simulink model "IEEE9Buses"  (R2024b)
settings: Solver=FixedStepAuto  StartTime=0  StopTime=5  FixedStep=1e-6  RelTol=1e-3
values from neighbouring files (symbols this model uses):
  SG_D_1_D = 0.01056    [SG9_parameters.m]
  SG_D_1_EnableSaturation = 0    [SG9_parameters.m]
  SG_D_1_f0 = 60    [SG9_parameters.m]
  SG_D_1_H = 7.5    [SG9_parameters.m]
  SG_D_1_K_A = 20    [SG9_parameters.m]
  SG_D_1_K_E = 1.000000e+1    (= 10)    [SG9_parameters.m]
  SG_D_1_K_F = 2.363    [SG9_parameters.m]
  SG_D_1_K_s = 5    [SG9_parameters.m]
  SG_D_1_R_a = 0.001088    [SG9_parameters.m]
  SG_D_1_S_A = 1    [SG9_parameters.m]
  SG_D_1_S_B = 0.103    [SG9_parameters.m]
  SG_D_1_S_N = 10.659857    [SG9_parameters.m]
  SG_D_1_SpeedPara = 200    [SG9_parameters.m]
  SG_D_1_T_0 = 0.720173    [SG9_parameters.m]
  SG_D_1_T_1 = 0.3    [SG9_parameters.m]
  SG_D_1_T_2 = 0.05    [SG9_parameters.m]
  SG_D_1_T_3 = 0.02    [SG9_parameters.m]
  SG_D_1_T_4 = 0.005    [SG9_parameters.m]
  SG_D_1_T_A = 0.02    [SG9_parameters.m]
  SG_D_1_T_dd = 8.000000e+0    (= 8)    [SG9_parameters.m]
  SG_D_1_T_ddd = 0.04    [SG9_parameters.m]
  SG_D_1_T_E = 0.314    [SG9_parameters.m]
  SG_D_1_T_F = 0.35    [SG9_parameters.m]
  SG_D_1_T_qd = 0.8    [SG9_parameters.m]
  SG_D_1_T_qdd = 0.02    [SG9_parameters.m]
  SG_D_1_T_speed = 0.1    [SG9_parameters.m]
  SG_D_1_T_w = 0.5    [SG9_parameters.m]
  SG_D_1_V_ref = 1.990276    [SG9_parameters.m]
  SG_D_1_w_ref = 376.991118    [SG9_parameters.m]
  SG_D_1_x_d = 1.9    [SG9_parameters.m]
  SG_D_1_x_dd = 0.302    [SG9_parameters.m]
  SG_D_1_x_ddd = 0.204    [SG9_parameters.m]
  SG_D_1_x_l = 0.05    [SG9_parameters.m]
  SG_D_1_x_q = 1.3    [SG9_parameters.m]
  SG_D_1_x_qd = 0.5    [SG9_parameters.m]
  SG_D_1_x_qdd = 0.3    [SG9_parameters.m]
  SG_D_2_D = 0.01056    [SG9_parameters.m]
  SG_D_2_EnableSaturation = 0    [SG9_parameters.m]
  SG_D_2_f0 = 60    [SG9_parameters.m]
  SG_D_2_H = 7.5    [SG9_parameters.m]
  SG_D_2_K_A = 20    [SG9_parameters.m]
  SG_D_2_K_E = 1.000000e+1    (= 10)    [SG9_parameters.m]
  SG_D_2_K_F = 2.363    [SG9_parameters.m]
  SG_D_2_K_s = 0.5    [SG9_parameters.m]
  SG_D_2_R_a = 0.001088    [SG9_parameters.m]
  SG_D_2_S_A = 1    [SG9_parameters.m]
  SG_D_2_S_B = 0.103    [SG9_parameters.m]
  SG_D_2_S_N = 10.659857    [SG9_parameters.m]
  SG_D_2_SpeedPara = 200    [SG9_parameters.m]
  SG_D_2_T_0 = 1.632913    [SG9_parameters.m]
  SG_D_2_T_1 = 0.2    [SG9_parameters.m]
  SG_D_2_T_2 = 0.05    [SG9_parameters.m]
  SG_D_2_T_3 = 0.02    [SG9_parameters.m]
  SG_D_2_T_4 = 0.005    [SG9_parameters.m]
  SG_D_2_T_A = 0.02    [SG9_parameters.m]
  SG_D_2_T_dd = 8.000000e+0    (= 8)    [SG9_parameters.m]
  SG_D_2_T_ddd = 0.04    [SG9_parameters.m]
  SG_D_2_T_E = 0.314    [SG9_parameters.m]
  SG_D_2_T_F = 0.35    [SG9_parameters.m]
  SG_D_2_T_qd = 0.8    [SG9_parameters.m]
  SG_D_2_T_qdd = 0.02    [SG9_parameters.m]
  SG_D_2_T_speed = 0.1    [SG9_parameters.m]
  SG_D_2_T_w = 0.5    [SG9_parameters.m]
  SG_D_2_V_ref = 2.662631    [SG9_parameters.m]
  SG_D_2_w_ref = 376.991118    [SG9_parameters.m]
  SG_D_2_x_d = 1.9    [SG9_parameters.m]
  SG_D_2_x_dd = 0.302    [SG9_parameters.m]
  SG_D_2_x_ddd = 0.204    [SG9_parameters.m]
  SG_D_2_x_l = 0.05    [SG9_parameters.m]
  SG_D_2_x_q = 1.3    [SG9_parameters.m]
  SG_D_2_x_qd = 0.5    [SG9_parameters.m]
  SG_D_2_x_qdd = 0.3    [SG9_parameters.m]
  SG_D_3_D = 0.01056    [SG9_parameters.m]
  SG_D_3_EnableSaturation = 0    [SG9_parameters.m]
  SG_D_3_f0 = 60    [SG9_parameters.m]
  SG_D_3_H = 7.5    [SG9_parameters.m]
  SG_D_3_K_A = 20    [SG9_parameters.m]
  SG_D_3_K_E = 1.000000e+1    (= 10)    [SG9_parameters.m]
  SG_D_3_K_F = 2.363    [SG9_parameters.m]
  SG_D_3_K_s = 0.5    [SG9_parameters.m]
  SG_D_3_R_a = 0.001088    [SG9_parameters.m]
  SG_D_3_S_A = 1    [SG9_parameters.m]
  SG_D_3_S_B = 0.103    [SG9_parameters.m]
  SG_D_3_S_N = 10.659857    [SG9_parameters.m]
  SG_D_3_SpeedPara = 200    [SG9_parameters.m]
  SG_D_3_T_0 = 0.850788    [SG9_parameters.m]
  SG_D_3_T_1 = 0.2    [SG9_parameters.m]
  SG_D_3_T_2 = 0.05    [SG9_parameters.m]
  SG_D_3_T_3 = 0.02    [SG9_parameters.m]
  SG_D_3_T_4 = 0.005    [SG9_parameters.m]
  SG_D_3_T_A = 0.02    [SG9_parameters.m]
  SG_D_3_T_dd = 8.000000e+0    (= 8)    [SG9_parameters.m]
  SG_D_3_T_ddd = 0.04    [SG9_parameters.m]
  SG_D_3_T_E = 0.314    [SG9_parameters.m]
  SG_D_3_T_F = 0.35    [SG9_parameters.m]
  SG_D_3_T_qd = 0.8    [SG9_parameters.m]
  SG_D_3_T_qdd = 0.02    [SG9_parameters.m]
  SG_D_3_T_speed = 0.1    [SG9_parameters.m]
  SG_D_3_T_w = 0.5    [SG9_parameters.m]
  SG_D_3_V_ref = 1.915682    [SG9_parameters.m]
  SG_D_3_w_ref = 376.991118    [SG9_parameters.m]
  SG_D_3_x_d = 1.9    [SG9_parameters.m]
  SG_D_3_x_dd = 0.302    [SG9_parameters.m]
  SG_D_3_x_ddd = 0.204    [SG9_parameters.m]
  SG_D_3_x_l = 0.05    [SG9_parameters.m]
  SG_D_3_x_q = 1.3    [SG9_parameters.m]
  SG_D_3_x_qd = 0.5    [SG9_parameters.m]
  SG_D_3_x_qdd = 0.3    [SG9_parameters.m]
(part 5 of 9)

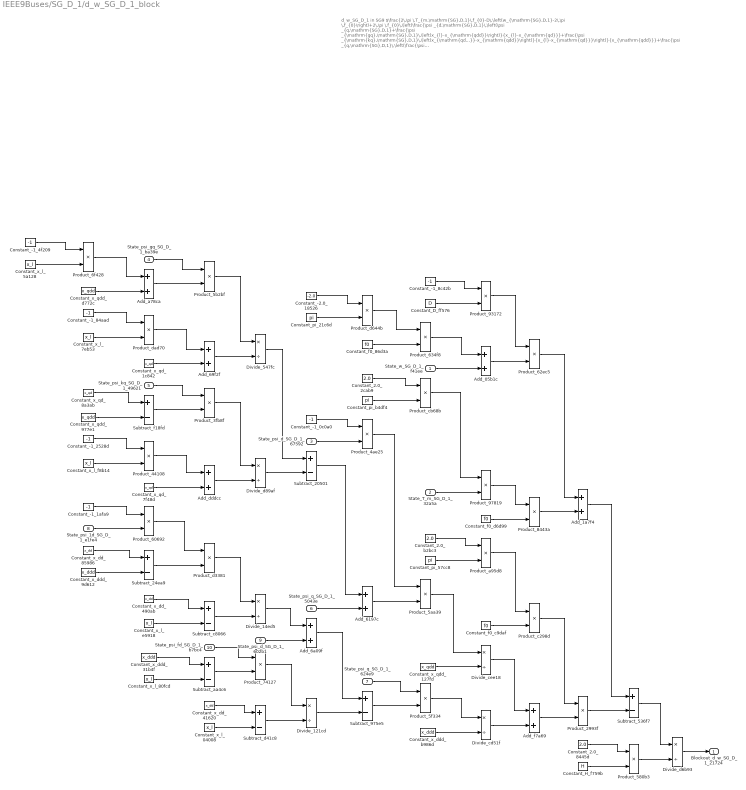
== system IEEE9Buses/SG_D_1/d_w_SG_D_1_block ==
  note: d_w_SG_D_1 in SG9
      | $\frac{2\,\pi \,T_{m,\mathrm{SG},D,1}\,f_{0}-D\,\left(w_{\mathrm{SG},D,1}-2\,\pi \,f_{0}\right)+2\,\pi \,f_{0}\,\left(\frac{\psi _{d,\mathrm{SG},D,1}\,\left(\psi _{q,\mathrm{SG},D,1}+\frac{\psi _{\mathrm{gq},\mathrm{SG},D,1}\,\left(x_{l}-x_{\mathrm{qdd}}\right)}{x_{l}-x_{\mathrm{qd}}}+\frac{\psi _{\mathrm{kq},\mathrm{SG},D,1}\,\left(x_{\mathrm{qd}}-x_{\mathrm{qdd}}\right)}{x_{l}-x_{\mathrm{qd}}}\right)}{x_{\mathrm{qdd}}}+\frac{\psi _{q,\mathrm{SG},D,1}\,\left(\frac{\psi _{\mathrm{1d},\mathrm{SG},D,1}\,\left(x_{\mathrm{dd}}-x_{\mathrm{ddd}}\right)}{x_{\mathrm{dd}}-x_{l}}-\psi _{d,\mathrm{SG},D,1}+\frac{\psi _{\mathrm{fd},\mathrm{SG},D,1}\,\left(x_{\mathrm{ddd}}-x_{l}\right)}{x_{\mathrm{dd}}-x_{l}}\right)}{x_{\mathrm{ddd}}}\right)}{2\,H}$
      | Automatically generated on 2025-09-12 21:31:18 .
  State_w_SG_D_1_f41ee : Inport
  State_T_m_SG_D_1_32a5a : Inport  Port=2
  State_psi_d_SG_D_1_67592 : Inport  Port=3
  State_psi_gq_SG_D_1_ba39e : Inport  Port=4
  State_psi_kq_SG_D_1_49621 : Inport  Port=5
  State_psi_q_SG_D_1_5043e : Inport  Port=6
  State_psi_q_SG_D_1_624e9 : Inport  Port=7
  State_psi_1d_SG_D_1_e1fe4 : Inport  Port=8
  State_psi_d_SG_D_1_602b1 : Inport  Port=9
  State_psi_fd_SG_D_1_b7bc4 : Inport  Port=10
  Add_05b1c : Sum
  Add_1a7f4 : Sum
  Add_6197c : Sum
  Add_69f2f : Sum
  Add_6a09f : Sum
  Add_a78ca : Sum
  Add_dddcc : Sum
  Add_f7a69 : Sum
  Constant_-1_0c0a0 : Constant  Value=-1
  Constant_-1_1afa9 : Constant  Value=-1
  Constant_-1_2528d : Constant  Value=-1
  Constant_-1_4f209 : Constant  Value=-1
  Constant_-1_84aad : Constant  Value=-1
  Constant_-1_8c42b : Constant  Value=-1
  Constant_-2.0_18526 : Constant  Value=-2.0
  Constant_2.0_2cab9 : Constant  Value=2.0
  Constant_2.0_8445d : Constant  Value=2.0
  Constant_2.0_b2bc3 : Constant  Value=2.0
  Constant_D_ff576 : Constant  Value=D
  Constant_H_f759b : Constant  Value=H
  Constant_f0_86d3a : Constant  Value=f0
  Constant_f0_c9daf : Constant  Value=f0
  Constant_f0_d6d99 : Constant  Value=f0
  Constant_pi_21c6d : Constant  Value=pi
  Constant_pi_57cc8 : Constant  Value=pi
  Constant_pi_b4df4 : Constant  Value=pi
  Constant_x_dd_41620 : Constant  Value=x_dd
  Constant_x_dd_490ab : Constant  Value=x_dd
  Constant_x_dd_85986 : Constant  Value=x_dd
  Constant_x_ddd_31b4f : Constant  Value=x_ddd
  Constant_x_ddd_9d612 : Constant  Value=x_ddd
  Constant_x_ddd_b986d : Constant  Value=x_ddd
  Constant_x_l_04008 : Constant  Value=x_l
  Constant_x_l_5a128 : Constant  Value=x_l
  Constant_x_l_7eb53 : Constant  Value=x_l
  Constant_x_l_80fcd : Constant  Value=x_l
  Constant_x_l_e5918 : Constant  Value=x_l
  Constant_x_l_f8b14 : Constant  Value=x_l
  Constant_x_qd_1c842 : Constant  Value=x_qd
  Constant_x_qd_7f48d : Constant  Value=x_qd
  Constant_x_qd_8a3ab : Constant  Value=x_qd
  Constant_x_qdd_127fd : Constant  Value=x_qdd
  Constant_x_qdd_977e1 : Constant  Value=x_qdd
  Constant_x_qdd_d772c : Constant  Value=x_qdd
  Divide_121cd : Product  Inputs=*/
  Divide_14ed5 : Product  Inputs=*/
  Divide_547fc : Product  Inputs=*/
  Divide_cd51f : Product  Inputs=*/
  Divide_cee18 : Product  Inputs=*/
  Divide_d6b93 : Product  Inputs=*/
  Divide_d89af : Product  Inputs=*/
  Product_2993f : Product
  Product_3fb8f : Product
  Product_{44108,60692,74127,93172,97819} (5 alike) : Product
  Product_4ae25 : Product
  Product_580b3 : Product
  Product_5aa39 : Product
  Product_5b2bf : Product
  Product_5f334 : Product
  Product_62ec5 : Product
  Product_634f8 : Product
  Product_6f428 : Product
  Product_8443a : Product
  Product_a95d8 : Product
  Product_c298d : Product
  Product_cb68b : Product
  Product_d3381 : Product
  Product_d644b : Product
  Product_dad70 : Product
  Subtract_20501 : Sum  Inputs=+-
  Subtract_24ea9 : Sum  Inputs=+-
  Subtract_536f7 : Sum  Inputs=+-
  Subtract_975e5 : Sum  Inputs=+-
  Subtract_aa4c6 : Sum  Inputs=+-
  Subtract_c8066 : Sum  Inputs=+-
  Subtract_d41c8 : Sum  Inputs=+-
  Subtract_f18fd : Sum  Inputs=+-
  Blockout_d_w_SG_D_1_21724 : Outport
  wires:
  Product_634f8/1 -> Add_05b1c/1
  Constant_-1_4f209/1 -> Product_6f428/1
  Constant_pi_b4df4/1 -> Product_cb68b/2
  Constant_x_qdd_d772c/1 -> Add_a78ca/2
  Constant_x_l_5a128/1 -> Product_6f428/2
  Product_6f428/1 -> Add_a78ca/1
  Constant_x_qd_8a3ab/1 -> Subtract_f18fd/1
  Constant_-1_84aad/1 -> Product_dad70/1
  Product_d644b/1 -> Product_634f8/1
  Constant_x_qdd_977e1/1 -> Subtract_f18fd/2
  State_psi_q_SG_D_1_624e9/1 -> Product_5f334/1
  Constant_x_l_7eb53/1 -> Product_dad70/2
  Constant_-1_2528d/1 -> Product_44108/1
  Constant_x_l_f8b14/1 -> Product_44108/2
  Constant_-1_1afa9/1 -> Product_60692/1
  Product_dad70/1 -> Add_69f2f/1
  State_psi_1d_SG_D_1_e1fe4/1 -> Product_60692/2
  Constant_x_dd_85986/1 -> Subtract_24ea9/1
  Subtract_f18fd/1 -> Product_3fb8f/2
  Constant_x_ddd_9d612/1 -> Subtract_24ea9/2
  State_psi_gq_SG_D_1_ba39e/1 -> Product_5b2bf/1
  Product_4ae25/1 -> Product_5aa39/1
  Add_a78ca/1 -> Product_5b2bf/2
  Constant_x_qd_1c842/1 -> Add_69f2f/2
  State_psi_kq_SG_D_1_49621/1 -> Product_3fb8f/1
  Constant_f0_86d3a/1 -> Product_634f8/2
  Product_44108/1 -> Add_dddcc/1
  Constant_x_dd_490ab/1 -> Subtract_c8066/1
  Constant_x_qd_7f48d/1 -> Add_dddcc/2
  Product_60692/1 -> Product_d3381/1
  Subtract_24ea9/1 -> Product_d3381/2
  Constant_x_l_e5918/1 -> Subtract_c8066/2
  Constant_x_ddd_31b4f/1 -> Subtract_aa4c6/1
  Constant_x_l_80fcd/1 -> Subtract_aa4c6/2
  State_w_SG_D_1_f41ee/1 -> Add_05b1c/2
  Divide_cee18/1 -> Add_f7a69/1
  Constant_-1_8c42b/1 -> Product_93172/1
  Product_5b2bf/1 -> Divide_547fc/1
  Add_05b1c/1 -> Product_62ec5/2
  Divide_547fc/1 -> Subtract_20501/1
  Add_69f2f/1 -> Divide_547fc/2
  Constant_pi_21c6d/1 -> Product_d644b/2
  Product_3fb8f/1 -> Divide_d89af/1
  Add_dddcc/1 -> Divide_d89af/2
  Product_d3381/1 -> Divide_14ed5/1
  Divide_14ed5/1 -> Add_6a09f/1
  Subtract_c8066/1 -> Divide_14ed5/2
  State_psi_fd_SG_D_1_b7bc4/1 -> Product_74127/1
  Subtract_aa4c6/1 -> Product_74127/2
  Constant_x_dd_41620/1 -> Subtract_d41c8/1
  Constant_x_l_04008/1 -> Subtract_d41c8/2
  Divide_d89af/1 -> Subtract_20501/2
  Constant_2.0_2cab9/1 -> Product_cb68b/1
  State_psi_d_SG_D_1_602b1/1 -> Add_6a09f/2
  Product_74127/1 -> Divide_121cd/1
  Subtract_d41c8/1 -> Divide_121cd/2
  Constant_-2.0_18526/1 -> Product_d644b/1
  Constant_-1_0c0a0/1 -> Product_4ae25/1
  State_psi_d_SG_D_1_67592/1 -> Product_4ae25/2
  Subtract_20501/1 -> Add_6197c/1
  Subtract_975e5/1 -> Product_5f334/2
  State_psi_q_SG_D_1_5043e/1 -> Add_6197c/2
  Add_6a09f/1 -> Subtract_975e5/1
  Divide_121cd/1 -> Subtract_975e5/2
  Add_6197c/1 -> Product_5aa39/2
  Constant_D_ff576/1 -> Product_93172/2
  Product_cb68b/1 -> Product_97819/1
  State_T_m_SG_D_1_32a5a/1 -> Product_97819/2
  Constant_2.0_b2bc3/1 -> Product_a95d8/1
  Constant_pi_57cc8/1 -> Product_a95d8/2
  Product_5aa39/1 -> Divide_cee18/1
  Constant_x_qdd_127fd/1 -> Divide_cee18/2
  Product_5f334/1 -> Divide_cd51f/1
  Constant_x_ddd_b986d/1 -> Divide_cd51f/2
  Product_93172/1 -> Product_62ec5/1
  Product_97819/1 -> Product_8443a/1
  Constant_f0_d6d99/1 -> Product_8443a/2
  Product_a95d8/1 -> Product_c298d/1
  Constant_f0_c9daf/1 -> Product_c298d/2
  Divide_cd51f/1 -> Add_f7a69/2
  Product_62ec5/1 -> Add_1a7f4/1
  Product_8443a/1 -> Add_1a7f4/2
  Product_c298d/1 -> Product_2993f/1
  Add_f7a69/1 -> Product_2993f/2
  Add_1a7f4/1 -> Subtract_536f7/1
  Product_2993f/1 -> Subtract_536f7/2
  Constant_2.0_8445d/1 -> Product_580b3/1
  Constant_H_f759b/1 -> Product_580b3/2
  Subtract_536f7/1 -> Divide_d6b93/1
  Product_580b3/1 -> Divide_d6b93/2
  Divide_d6b93/1 -> Blockout_d_w_SG_D_1_21724/1

== system IEEE9Buses/SG_D_1/i_d_SG_D_1_block ==
  note: i_d_SG_D_1 in SG9
      | $\frac{\sin\left(\theta _{\mathrm{SG},D,1}\right)\,\left(\frac{\psi _{\mathrm{1d},\mathrm{SG},D,1}\,\left(x_{\mathrm{dd}}-x_{\mathrm{ddd}}\right)}{x_{\mathrm{dd}}-x_{l}}-\psi _{d,\mathrm{SG},D,1}+\frac{\psi _{\mathrm{fd},\mathrm{SG},D,1}\,\left(x_{\mathrm{ddd}}-x_{l}\right)}{x_{\mathrm{dd}}-x_{l}}\right)}{x_{\mathrm{ddd}}}-\frac{\cos\left(\theta _{\mathrm{SG},D,1}\right)\,\left(\psi _{q,\mathrm{SG},D,1}+\frac{\psi _{\mathrm{gq},\mathrm{SG},D,1}\,\left(x_{l}-x_{\mathrm{qdd}}\right)}{x_{l}-x_{\mathrm{qd}}}+\frac{\psi _{\mathrm{kq},\mathrm{SG},D,1}\,\left(x_{\mathrm{qd}}-x_{\mathrm{qdd}}\right)}{x_{l}-x_{\mathrm{qd}}}\right)}{x_{\mathrm{qdd}}}$
      | Automatically generated on 2025-09-12 21:31:40 .
  State_psi_gq_SG_D_1_16d47 : Inport
  State_psi_kq_SG_D_1_e3ffd : Inport  Port=2
  State_psi_q_SG_D_1_6d935 : Inport  Port=3
  State_theta_SG_D_1_f0743 : Inport  Port=4
  State_psi_1d_SG_D_1_2c6db : Inport  Port=5
  State_psi_d_SG_D_1_87c65 : Inport  Port=6
  State_psi_fd_SG_D_1_32fec : Inport  Port=7
  State_theta_SG_D_1_03b3d : Inport  Port=8
  Add_0e858 : Sum
  Add_4610b : Sum
  Add_7770e : Sum
  Add_d2edc : Sum
  Add_d8f47 : Sum
  Constant_-1_131e8 : Constant  Value=-1
  Constant_-1_32ee8 : Constant  Value=-1
  Constant_-1_419e7 : Constant  Value=-1
  Constant_-1_52bf1 : Constant  Value=-1
  Constant_-1_ea77c : Constant  Value=-1
  Constant_x_dd_0537a : Constant  Value=x_dd
  Constant_x_dd_97a3f : Constant  Value=x_dd
  Constant_x_dd_feb13 : Constant  Value=x_dd
  Constant_x_ddd_1be8c : Constant  Value=x_ddd
  Constant_x_ddd_28448 : Constant  Value=x_ddd
  Constant_x_ddd_b6170 : Constant  Value=x_ddd
  Constant_x_l_23288 : Constant  Value=x_l
  Constant_x_l_57c7a : Constant  Value=x_l
  Constant_x_l_6da32 : Constant  Value=x_l
  Constant_x_l_7756f : Constant  Value=x_l
  Constant_x_l_7edcb : Constant  Value=x_l
  Constant_x_l_90c3f : Constant  Value=x_l
  Constant_x_qd_0c1e5 : Constant  Value=x_qd
  Constant_x_qd_4a689 : Constant  Value=x_qd
  Constant_x_qd_832d5 : Constant  Value=x_qd
  Constant_x_qdd_149fe : Constant  Value=x_qdd
  Constant_x_qdd_5abe7 : Constant  Value=x_qdd
  Constant_x_qdd_fcf28 : Constant  Value=x_qdd
  Divide_03f77 : Product  Inputs=*/
  Divide_182f0 : Product  Inputs=*/
  Divide_3d8fe : Product  Inputs=*/
  Divide_b82b4 : Product  Inputs=*/
  Divide_dd0cc : Product  Inputs=*/
  Divide_fa6c8 : Product  Inputs=*/
  MathFunc_cos_619ce : Trigonometry  Operator=cos
  MathFunc_sin_33313 : Trigonometry
  Product_060bb : Product
  Product_2162b : Product
  Product_54330 : Product
  Product_56fc4 : Product
  Product_79475 : Product
  Product_9e944 : Product
  Product_b429e : Product
  Product_bcdeb : Product
  Product_e3228 : Product
  Product_e561b : Product
  Product_ed3ce : Product
  Subtract_04101 : Sum  Inputs=+-
  Subtract_17c36 : Sum  Inputs=+-
  Subtract_32416 : Sum  Inputs=+-
  Subtract_778c2 : Sum  Inputs=+-
  Subtract_7dc08 : Sum  Inputs=+-
  Subtract_9f997 : Sum  Inputs=+-
  Subtract_b4766 : Sum  Inputs=+-
  Subtract_dd9ee : Sum  Inputs=+-
  Blockout_i_d_SG_D_1_3e23c : Outport
  wires:
  Constant_-1_52bf1/1 -> Product_56fc4/1
  Constant_x_l_7edcb/1 -> Product_56fc4/2
  Constant_x_ddd_28448/1 -> Subtract_dd9ee/2
  Product_56fc4/1 -> Add_d8f47/1
  Constant_x_qdd_5abe7/1 -> Subtract_7dc08/2
  Constant_x_l_90c3f/1 -> Product_54330/2
  Constant_x_qd_0c1e5/1 -> Add_d2edc/2
  Constant_x_qdd_fcf28/1 -> Add_d8f47/2
  Constant_x_qd_4a689/1 -> Subtract_7dc08/1
  MathFunc_cos_619ce/1 -> Product_bcdeb/2
  Constant_-1_419e7/1 -> Product_54330/1
  Constant_-1_131e8/1 -> Product_9e944/1
  Subtract_17c36/1 -> Blockout_i_d_SG_D_1_3e23c/1
  Constant_x_l_7756f/1 -> Product_9e944/2
  Divide_182f0/1 -> Subtract_778c2/1
  State_psi_gq_SG_D_1_16d47/1 -> Product_ed3ce/1
  Subtract_b4766/1 -> Product_e561b/2
  Add_d8f47/1 -> Product_ed3ce/2
  Divide_fa6c8/1 -> Add_4610b/1
  Product_54330/1 -> Add_7770e/1
  Constant_x_qd_832d5/1 -> Add_7770e/2
  State_psi_kq_SG_D_1_e3ffd/1 -> Product_e3228/1
  Add_4610b/1 -> Subtract_04101/1
  Add_7770e/1 -> Divide_182f0/2
  Subtract_7dc08/1 -> Product_e3228/2
  Product_9e944/1 -> Add_d2edc/1
  Constant_-1_ea77c/1 -> Product_79475/1
  State_psi_1d_SG_D_1_2c6db/1 -> Product_79475/2
  Constant_x_dd_feb13/1 -> Subtract_dd9ee/1
  Product_ed3ce/1 -> Divide_182f0/1
  Product_2162b/1 -> Divide_03f77/1
  Subtract_dd9ee/1 -> Product_060bb/2
  Product_e3228/1 -> Divide_b82b4/1
  Product_79475/1 -> Product_060bb/1
  Add_d2edc/1 -> Divide_b82b4/2
  Constant_x_dd_0537a/1 -> Subtract_32416/1
  Subtract_778c2/1 -> Add_0e858/1
  Constant_x_l_57c7a/1 -> Subtract_32416/2
  Constant_x_ddd_b6170/1 -> Subtract_b4766/1
  Constant_x_l_6da32/1 -> Subtract_b4766/2
  Divide_03f77/1 -> Subtract_17c36/2
  Divide_b82b4/1 -> Subtract_778c2/2
  State_theta_SG_D_1_f0743/1 -> MathFunc_cos_619ce/1
  Product_060bb/1 -> Divide_fa6c8/1
  Subtract_32416/1 -> Divide_fa6c8/2
  State_theta_SG_D_1_03b3d/1 -> MathFunc_sin_33313/1
  State_psi_fd_SG_D_1_32fec/1 -> Product_e561b/1
  Constant_x_dd_97a3f/1 -> Subtract_9f997/1
  Constant_x_l_23288/1 -> Subtract_9f997/2
  State_psi_q_SG_D_1_6d935/1 -> Add_0e858/2
  State_psi_d_SG_D_1_87c65/1 -> Add_4610b/2
  Constant_x_ddd_1be8c/1 -> Divide_03f77/2
  MathFunc_sin_33313/1 -> Product_2162b/2
  Product_e561b/1 -> Divide_dd0cc/1
  Constant_-1_32ee8/1 -> Product_b429e/1
  Subtract_9f997/1 -> Divide_dd0cc/2
  Add_0e858/1 -> Product_b429e/2
  Divide_dd0cc/1 -> Subtract_04101/2
  Product_b429e/1 -> Product_bcdeb/1
  Subtract_04101/1 -> Product_2162b/1
  Constant_x_qdd_149fe/1 -> Divide_3d8fe/2
  Product_bcdeb/1 -> Divide_3d8fe/1
  Divide_3d8fe/1 -> Subtract_17c36/1

== system IEEE9Buses/SG_D_1/i_q_SG_D_1_block ==
  note: i_q_SG_D_1 in SG9
      | $-\frac{\sin\left(\theta _{\mathrm{SG},D,1}\right)\,\left(\psi _{q,\mathrm{SG},D,1}+\frac{\psi _{\mathrm{gq},\mathrm{SG},D,1}\,\left(x_{l}-x_{\mathrm{qdd}}\right)}{x_{l}-x_{\mathrm{qd}}}+\frac{\psi _{\mathrm{kq},\mathrm{SG},D,1}\,\left(x_{\mathrm{qd}}-x_{\mathrm{qdd}}\right)}{x_{l}-x_{\mathrm{qd}}}\right)}{x_{\mathrm{qdd}}}-\frac{\cos\left(\theta _{\mathrm{SG},D,1}\right)\,\left(\frac{\psi _{\mathrm{1d},\mathrm{SG},D,1}\,\left(x_{\mathrm{dd}}-x_{\mathrm{ddd}}\right)}{x_{\mathrm{dd}}-x_{l}}-\psi _{d,\mathrm{SG},D,1}+\frac{\psi _{\mathrm{fd},\mathrm{SG},D,1}\,\left(x_{\mathrm{ddd}}-x_{l}\right)}{x_{\mathrm{dd}}-x_{l}}\right)}{x_{\mathrm{ddd}}}$
      | Automatically generated on 2025-09-12 21:31:43 .
  State_psi_gq_SG_D_1_ea88a : Inport
  State_psi_kq_SG_D_1_bbf34 : Inport  Port=2
  State_psi_q_SG_D_1_2c971 : Inport  Port=3
  State_theta_SG_D_1_dbec2 : Inport  Port=4
  State_psi_1d_SG_D_1_2130a : Inport  Port=5
  State_psi_d_SG_D_1_6fa4d : Inport  Port=6
  State_psi_fd_SG_D_1_79f47 : Inport  Port=7
  State_theta_SG_D_1_fb79e : Inport  Port=8
  Add_47eff : Sum
  Add_4c55d : Sum
  Add_4ffe0 : Sum
  Add_95e4b : Sum
  Add_cf20e : Sum
  Add_d3f92 : Sum
  Constant_-1_62bcf : Constant  Value=-1
  Constant_-1_a9bb9 : Constant  Value=-1
  Constant_-1_d820a : Constant  Value=-1
  Constant_-1_ef529 : Constant  Value=-1
  Constant_-1_fab4c : Constant  Value=-1
  Constant_x_dd_1cb78 : Constant  Value=x_dd
  Constant_x_dd_226a4 : Constant  Value=x_dd
  Constant_x_dd_8a0da : Constant  Value=x_dd
  Constant_x_ddd_03912 : Constant  Value=x_ddd
  Constant_x_ddd_2a32c : Constant  Value=x_ddd
  Constant_x_ddd_da055 : Constant  Value=x_ddd
  Constant_x_l_3e93c : Constant  Value=x_l
  Constant_x_l_3fde4 : Constant  Value=x_l
  Constant_x_l_52f30 : Constant  Value=x_l
  Constant_x_l_9f34b : Constant  Value=x_l
  Constant_x_l_a8bb7 : Constant  Value=x_l
  Constant_x_l_ae924 : Constant  Value=x_l
  Constant_x_qd_0a82d : Constant  Value=x_qd
  Constant_x_qd_bd232 : Constant  Value=x_qd
  Constant_x_qd_cfcb5 : Constant  Value=x_qd
  Constant_x_qdd_5c57a : Constant  Value=x_qdd
  Constant_x_qdd_62b62 : Constant  Value=x_qdd
  Constant_x_qdd_d360d : Constant  Value=x_qdd
  Divide_030c8 : Product  Inputs=*/
  Divide_0be4c : Product  Inputs=*/
  Divide_3da13 : Product  Inputs=*/
  Divide_46592 : Product  Inputs=*/
  Divide_bebe2 : Product  Inputs=*/
  Divide_d4446 : Product  Inputs=*/
  MathFunc_cos_61b8c : Trigonometry  Operator=cos
  MathFunc_sin_2edd4 : Trigonometry
  Product_10577 : Product
  Product_345d6 : Product
  Product_734fb : Product
  Product_7ee05 : Product
  Product_833e5 : Product
  Product_86d2a : Product
  Product_914ef : Product
  Product_93beb : Product
  Product_99182 : Product
  Product_dc880 : Product
  Product_e0634 : Product
  Subtract_06b7f : Sum  Inputs=+-
  Subtract_1796b : Sum  Inputs=+-
  Subtract_5f76f : Sum  Inputs=+-
  Subtract_62225 : Sum  Inputs=+-
  Subtract_69ee0 : Sum  Inputs=+-
  Subtract_72da9 : Sum  Inputs=+-
  Subtract_fb50c : Sum  Inputs=+-
  Blockout_i_q_SG_D_1_e8e0f : Outport
  wires:
  State_theta_SG_D_1_fb79e/1 -> MathFunc_cos_61b8c/1
  State_psi_fd_SG_D_1_79f47/1 -> Product_93beb/1
  Constant_-1_ef529/1 -> Product_86d2a/1
  Constant_x_l_9f34b/1 -> Product_86d2a/2
  Subtract_06b7f/1 -> Product_93beb/2
  Constant_x_l_3fde4/1 -> Subtract_1796b/2
  Product_86d2a/1 -> Add_47eff/1
  Constant_x_qdd_d360d/1 -> Add_47eff/2
  Constant_x_qd_cfcb5/1 -> Subtract_5f76f/1
  Constant_x_qdd_5c57a/1 -> Divide_bebe2/2
  MathFunc_sin_2edd4/1 -> Product_833e5/2
  Constant_-1_fab4c/1 -> Product_345d6/1
  Constant_x_qdd_62b62/1 -> Subtract_5f76f/2
  Add_cf20e/1 -> Product_dc880/2
  Product_10577/1 -> Divide_0be4c/1
  Constant_x_l_a8bb7/1 -> Product_345d6/2
  Constant_-1_a9bb9/1 -> Product_734fb/1
  Constant_x_l_ae924/1 -> Product_734fb/2
  State_psi_gq_SG_D_1_ea88a/1 -> Product_10577/1
  Add_47eff/1 -> Product_10577/2
  Divide_3da13/1 -> Add_4c55d/1
  Product_345d6/1 -> Add_d3f92/1
  Divide_bebe2/1 -> Add_95e4b/1
  Constant_x_qd_bd232/1 -> Add_d3f92/2
  State_psi_kq_SG_D_1_bbf34/1 -> Product_914ef/1
  Add_4c55d/1 -> Subtract_fb50c/1
  Subtract_5f76f/1 -> Product_914ef/2
  Divide_0be4c/1 -> Subtract_62225/1
  Add_d3f92/1 -> Divide_0be4c/2
  Product_734fb/1 -> Add_4ffe0/1
  Constant_x_qd_0a82d/1 -> Add_4ffe0/2
  Constant_-1_d820a/1 -> Product_99182/1
  MathFunc_cos_61b8c/1 -> Product_e0634/2
  Product_93beb/1 -> Divide_46592/1
  State_psi_1d_SG_D_1_2130a/1 -> Product_99182/2
  Constant_x_l_52f30/1 -> Subtract_72da9/2
  Constant_x_dd_226a4/1 -> Subtract_69ee0/1
  Divide_46592/1 -> Subtract_fb50c/2
  Constant_x_ddd_2a32c/1 -> Subtract_69ee0/2
  Product_e0634/1 -> Divide_d4446/1
  Product_914ef/1 -> Divide_030c8/1
  Product_99182/1 -> Product_7ee05/1
  Add_4ffe0/1 -> Divide_030c8/2
  Subtract_69ee0/1 -> Product_7ee05/2
  State_psi_d_SG_D_1_6fa4d/1 -> Add_4c55d/2
  Constant_x_dd_1cb78/1 -> Subtract_1796b/1
  Constant_x_ddd_da055/1 -> Subtract_06b7f/1
  Constant_x_l_3e93c/1 -> Subtract_06b7f/2
  Divide_d4446/1 -> Add_95e4b/2
  Divide_030c8/1 -> Subtract_62225/2
  State_theta_SG_D_1_dbec2/1 -> MathFunc_sin_2edd4/1
  Product_7ee05/1 -> Divide_3da13/1
  Subtract_1796b/1 -> Divide_3da13/2
  Constant_x_dd_8a0da/1 -> Subtract_72da9/1
  Subtract_62225/1 -> Add_cf20e/1
  State_psi_q_SG_D_1_2c971/1 -> Add_cf20e/2
  Subtract_72da9/1 -> Divide_46592/2
  Subtract_fb50c/1 -> Product_e0634/1
  Constant_-1_62bcf/1 -> Product_dc880/1
  Product_dc880/1 -> Product_833e5/1
  Product_833e5/1 -> Divide_bebe2/1
  Constant_x_ddd_03912/1 -> Divide_d4446/2
  Add_95e4b/1 -> Blockout_i_q_SG_D_1_e8e0f/1

== system IEEE9Buses/SG_D_1/theta_SG_D_1_out_block ==
  note: theta_SG_D_1_out in SG9
      | $\theta _{\mathrm{SG},D,1}$
      | Automatically generated on 2025-09-12 21:31:49 .
  State_theta_SG_D_1_c9f92 : Inport
  Blockout_theta_SG_D_1_out_eb1bc : Outport
  wires:
  State_theta_SG_D_1_c9f92/1 -> Blockout_theta_SG_D_1_out_eb1bc/1

== system IEEE9Buses/SG_D_1/w_SG_D_1_out_block ==
  note: w_SG_D_1_out in SG9
      | $w_{\mathrm{SG},D,1}$
      | Automatically generated on 2025-09-12 21:31:48 .
  State_w_SG_D_1_1a398 : Inport
  Blockout_w_SG_D_1_out_88950 : Outport
  wires:
  State_w_SG_D_1_1a398/1 -> Blockout_w_SG_D_1_out_88950/1

== system IEEE9Buses/SG_D_2/T_e_SG_D_2_block ==
  note: T_e_SG_D_2 in SG9
      | $-\frac{\psi _{d,\mathrm{SG},D,2}\,\left(\psi _{q,\mathrm{SG},D,2}+\frac{\psi _{\mathrm{gq},\mathrm{SG},D,2}\,\left(x_{l}-x_{\mathrm{qdd}}\right)}{x_{l}-x_{\mathrm{qd}}}+\frac{\psi _{\mathrm{kq},\mathrm{SG},D,2}\,\left(x_{\mathrm{qd}}-x_{\mathrm{qdd}}\right)}{x_{l}-x_{\mathrm{qd}}}\right)}{x_{\mathrm{qdd}}}-\frac{\psi _{q,\mathrm{SG},D,2}\,\left(\frac{\psi _{\mathrm{1d},\mathrm{SG},D,2}\,\left(x_{\mathrm{dd}}-x_{\mathrm{ddd}}\right)}{x_{\mathrm{dd}}-x_{l}}-\psi _{d,\mathrm{SG},D,2}+\frac{\psi _{\mathrm{fd},\mathrm{SG},D,2}\,\left(x_{\mathrm{ddd}}-x_{l}\right)}{x_{\mathrm{dd}}-x_{l}}\right)}{x_{\mathrm{ddd}}}$
      | Automatically generated on 2025-09-12 21:32:53 .
  State_psi_d_SG_D_2_c06bd : Inport
  State_psi_gq_SG_D_2_ad00d : Inport  Port=2
  State_psi_kq_SG_D_2_a60cc : Inport  Port=3
  State_psi_q_SG_D_2_25743 : Inport  Port=4
  State_psi_q_SG_D_2_3ca84 : Inport  Port=5
  State_psi_1d_SG_D_2_a239a : Inport  Port=6
  State_psi_d_SG_D_2_23d38 : Inport  Port=7
  State_psi_fd_SG_D_2_3f2f2 : Inport  Port=8
  Add_64332 : Sum
  Add_70402 : Sum
  Add_78f80 : Sum
  Add_7a74b : Sum
  Add_8b949 : Sum
  Add_de37c : Sum
  Constant_-1_3629c : Constant  Value=-1
  Constant_-1_64f25 : Constant  Value=-1
  Constant_-1_65f7b : Constant  Value=-1
  Constant_-1_9ba2c : Constant  Value=-1
  Constant_-1_cd5be : Constant  Value=-1
  Constant_x_dd_eef63 : Constant  Value=x_dd
  Constant_x_dd_f96bb : Constant  Value=x_dd
  Constant_x_dd_ff408 : Constant  Value=x_dd
  Constant_x_ddd_8cbf7 : Constant  Value=x_ddd
  Constant_x_ddd_8d60b : Constant  Value=x_ddd
  Constant_x_ddd_da575 : Constant  Value=x_ddd
  Constant_x_l_276ae : Constant  Value=x_l
  Constant_x_l_7bf73 : Constant  Value=x_l
  Constant_x_l_84997 : Constant  Value=x_l
  Constant_x_l_8ea2e : Constant  Value=x_l
  Constant_x_l_ab8c9 : Constant  Value=x_l
  Constant_x_l_d07bb : Constant  Value=x_l
  Constant_x_qd_ac5c7 : Constant  Value=x_qd
  Constant_x_qd_b5b9c : Constant  Value=x_qd
  Constant_x_qd_d42d4 : Constant  Value=x_qd
  Constant_x_qdd_7d47e : Constant  Value=x_qdd
  Constant_x_qdd_d8e56 : Constant  Value=x_qdd
  Constant_x_qdd_daf9f : Constant  Value=x_qdd
  Divide_022f5 : Product  Inputs=*/
  Divide_2ddae : Product  Inputs=*/
  Divide_4415f : Product  Inputs=*/
  Divide_63bd9 : Product  Inputs=*/
  Divide_9c904 : Product  Inputs=*/
  Divide_d760a : Product  Inputs=*/
  Product_051c6 : Product
  Product_1af36 : Product
  Product_22c43 : Product
  Product_3eaa0 : Product
  Product_4e0bc : Product
  Product_652af : Product
  Product_92ed0 : Product
  Product_ce9b5 : Product
  Product_d6b33 : Product
  Product_e99de : Product
  Product_fe9e2 : Product
  Subtract_0acff : Sum  Inputs=+-
  Subtract_2638b : Sum  Inputs=+-
  Subtract_5b6ef : Sum  Inputs=+-
  Subtract_7f17c : Sum  Inputs=+-
  Subtract_bf016 : Sum  Inputs=+-
  Subtract_bf4ab : Sum  Inputs=+-
  Subtract_e388c : Sum  Inputs=+-
  Blockout_T_e_SG_D_2_58459 : Outport
  wires:
  Constant_-1_65f7b/1 -> Product_92ed0/1
  Divide_63bd9/1 -> Subtract_bf4ab/1
  Constant_-1_64f25/1 -> Product_652af/1
  Constant_x_l_8ea2e/1 -> Product_652af/2
  Constant_x_qd_d42d4/1 -> Subtract_2638b/1
  Product_4e0bc/1 -> Divide_63bd9/1
  Product_652af/1 -> Add_7a74b/1
  Divide_022f5/1 -> Subtract_7f17c/2
  Constant_x_qdd_d8e56/1 -> Subtract_2638b/2
  Constant_x_qdd_7d47e/1 -> Divide_2ddae/2
  Constant_x_ddd_da575/1 -> Subtract_e388c/2
  Constant_x_qdd_daf9f/1 -> Add_7a74b/2
  Constant_x_l_276ae/1 -> Product_92ed0/2
  Constant_-1_3629c/1 -> Product_3eaa0/1
  Constant_x_l_7bf73/1 -> Product_3eaa0/2
  Constant_-1_cd5be/1 -> Product_fe9e2/1
  State_psi_1d_SG_D_2_a239a/1 -> Product_fe9e2/2
  Constant_x_dd_ff408/1 -> Subtract_e388c/1
  Divide_4415f/1 -> Subtract_bf4ab/2
  State_psi_gq_SG_D_2_ad00d/1 -> Product_4e0bc/1
  Add_7a74b/1 -> Product_4e0bc/2
  Subtract_bf4ab/1 -> Add_de37c/1
  Constant_x_dd_f96bb/1 -> Subtract_5b6ef/1
  Product_92ed0/1 -> Add_70402/1
  Product_051c6/1 -> Product_d6b33/1
  Constant_x_qd_b5b9c/1 -> Add_70402/2
  State_psi_kq_SG_D_2_a60cc/1 -> Product_22c43/1
  Subtract_2638b/1 -> Product_22c43/2
  Product_3eaa0/1 -> Add_78f80/1
  State_psi_q_SG_D_2_3ca84/1 -> Product_1af36/1
  Constant_x_qd_ac5c7/1 -> Add_78f80/2
  Product_fe9e2/1 -> Product_e99de/1
  Divide_d760a/1 -> Add_64332/2
  Subtract_e388c/1 -> Product_e99de/2
  Constant_x_l_84997/1 -> Subtract_5b6ef/2
  Constant_x_ddd_8cbf7/1 -> Subtract_bf016/1
  Constant_x_dd_eef63/1 -> Subtract_0acff/1
  Constant_x_l_d07bb/1 -> Subtract_bf016/2
  Add_64332/1 -> Blockout_T_e_SG_D_2_58459/1
  Add_70402/1 -> Divide_63bd9/2
  Product_22c43/1 -> Divide_4415f/1
  Product_d6b33/1 -> Divide_2ddae/1
  State_psi_d_SG_D_2_c06bd/1 -> Product_051c6/2
  Add_78f80/1 -> Divide_4415f/2
  Product_e99de/1 -> Divide_9c904/1
  Subtract_5b6ef/1 -> Divide_9c904/2
  Constant_x_l_ab8c9/1 -> Subtract_0acff/2
  State_psi_fd_SG_D_2_3f2f2/1 -> Product_ce9b5/1
  Constant_x_ddd_8d60b/1 -> Divide_d760a/2
  Product_1af36/1 -> Divide_d760a/1
  Subtract_bf016/1 -> Product_ce9b5/2
  Divide_9c904/1 -> Add_8b949/1
  State_psi_d_SG_D_2_23d38/1 -> Add_8b949/2
  Add_8b949/1 -> Subtract_7f17c/1
  Product_ce9b5/1 -> Divide_022f5/1
  Subtract_0acff/1 -> Divide_022f5/2
  Constant_-1_9ba2c/1 -> Product_051c6/1
  State_psi_q_SG_D_2_25743/1 -> Add_de37c/2
  Add_de37c/1 -> Product_d6b33/2
  Subtract_7f17c/1 -> Product_1af36/2
  Divide_2ddae/1 -> Add_64332/1

== system IEEE9Buses/SG_D_2/d_E_fd_SG_D_2_block ==
  note: d_E_fd_SG_D_2 in SG9
      | $\frac{V_{f,\mathrm{SG},D,2}-E_{\mathrm{fd},\mathrm{SG},D,2}\,K_{E}}{T_{E}}$
      | Automatically generated on 2025-09-12 21:32:37 .
  State_E_fd_SG_D_2_bb78e : Inport
  State_V_f_SG_D_2_155d9 : Inport  Port=2
  Add_9ae56 : Sum
  Constant_-1_79cf2 : Constant  Value=-1
  Constant_K_E_5f4a8 : Constant  Value=K_E
  Constant_T_E_3339a : Constant  Value=T_E
  Divide_90347 : Product  Inputs=*/
  Product_10f65 : Product
  Product_b6b34 : Product
  Blockout_d_E_fd_SG_D_2_eb42a : Outport
  wires:
  Constant_-1_79cf2/1 -> Product_10f65/1
  State_E_fd_SG_D_2_bb78e/1 -> Product_10f65/2
  Product_10f65/1 -> Product_b6b34/1
  Constant_K_E_5f4a8/1 -> Product_b6b34/2
  Product_b6b34/1 -> Add_9ae56/1
  Constant_T_E_3339a/1 -> Divide_90347/2
  State_V_f_SG_D_2_155d9/1 -> Add_9ae56/2
  Add_9ae56/1 -> Divide_90347/1
  Divide_90347/1 -> Blockout_d_E_fd_SG_D_2_eb42a/1

== system IEEE9Buses/SG_D_2/d_Px_1_SG_D_2_block ==
  note: d_Px_1_SG_D_2 in SG9
      | $\frac{w_{\mathrm{SG},D,2}-2\,\pi \,f_{0}}{T_{w}}-\frac{\mathrm{Px}_{1,\mathrm{SG},D,2}}{T_{w}}$
      | Automatically generated on 2025-09-12 21:32:39 .
  State_Px_1_SG_D_2_446b7 : Inport
  State_w_SG_D_2_2f75d : Inport  Port=2
  Add_df030 : Sum
  Add_fe7d1 : Sum
  Constant_-1_fea1e : Constant  Value=-1
  Constant_-2.0_a0b35 : Constant  Value=-2.0
  Constant_T_w_748d0 : Constant  Value=T_w
  Constant_T_w_94a1b : Constant  Value=T_w
  Constant_f0_5f790 : Constant  Value=f0
  Constant_pi_41c5d : Constant  Value=pi
  Divide_6f076 : Product  Inputs=*/
  Divide_6fe48 : Product  Inputs=*/
  Product_0f34a : Product
  Product_663e8 : Product
  Product_e785b : Product
  Blockout_d_Px_1_SG_D_2_5baad : Outport
  wires:
  Constant_-2.0_a0b35/1 -> Product_e785b/1
  State_w_SG_D_2_2f75d/1 -> Add_df030/2
  Constant_pi_41c5d/1 -> Product_e785b/2
  Product_e785b/1 -> Product_663e8/1
  Constant_f0_5f790/1 -> Product_663e8/2
  Constant_-1_fea1e/1 -> Product_0f34a/1
  State_Px_1_SG_D_2_446b7/1 -> Product_0f34a/2
  Product_663e8/1 -> Add_df030/1
  Product_0f34a/1 -> Divide_6fe48/1
  Constant_T_w_748d0/1 -> Divide_6fe48/2
  Add_df030/1 -> Divide_6f076/1
  Constant_T_w_94a1b/1 -> Divide_6f076/2
  Divide_6fe48/1 -> Add_fe7d1/1
  Divide_6f076/1 -> Add_fe7d1/2
  Add_fe7d1/1 -> Blockout_d_Px_1_SG_D_2_5baad/1

== system IEEE9Buses/SG_D_2/d_Px_2_SG_D_2_block ==
  note: d_Px_2_SG_D_2 in SG9
      | $\frac{\mathrm{Px}_{1,\mathrm{SG},D,2}-T_{2}\,\left(\frac{\mathrm{Px}_{1,\mathrm{SG},D,2}}{T_{w}}-\frac{w_{\mathrm{SG},D,2}-2\,\pi \,f_{0}}{T_{w}}\right)}{T_{1}}-\frac{\mathrm{Px}_{2,\mathrm{SG},D,2}}{T_{1}}$
      | Automatically generated on 2025-09-12 21:32:40 .
  State_Px_2_SG_D_2_f1aec : Inport
  State_Px_1_SG_D_2_41234 : Inport  Port=2
  State_Px_1_SG_D_2_b0ce9 : Inport  Port=3
  State_w_SG_D_2_4c038 : Inport  Port=4
  Add_18759 : Sum
  Add_77af2 : Sum
  Add_8d951 : Sum
  Add_93689 : Sum
  Constant_-1_1724e : Constant  Value=-1
  Constant_-1_d4b72 : Constant  Value=-1
  Constant_-2.0_1a60f : Constant  Value=-2.0
  Constant_T_1_35986 : Constant  Value=T_1
  Constant_T_1_cab14 : Constant  Value=T_1
  Constant_T_2_bd17f : Constant  Value=T_2
  Constant_T_w_ec2c5 : Constant  Value=T_w
  Constant_T_w_f7f42 : Constant  Value=T_w
  Constant_f0_7fafb : Constant  Value=f0
  Constant_pi_8bb9a : Constant  Value=pi
  Divide_56a39 : Product  Inputs=*/
  Divide_86fee : Product  Inputs=*/
  Divide_8e073 : Product  Inputs=*/
  Divide_9219e : Product  Inputs=*/
  Product_1a882 : Product
  Product_c813a : Product
  Product_cb5db : Product
  Product_e35d7 : Product
  Product_f39d7 : Product
  Blockout_d_Px_2_SG_D_2_af1ce : Outport
  wires:
  Constant_-1_d4b72/1 -> Product_f39d7/1
  Constant_-2.0_1a60f/1 -> Product_1a882/1
  Product_e35d7/1 -> Add_77af2/2
  State_w_SG_D_2_4c038/1 -> Add_93689/2
  Constant_pi_8bb9a/1 -> Product_1a882/2
  Product_1a882/1 -> Product_c813a/1
  State_Px_1_SG_D_2_b0ce9/1 -> Product_cb5db/2
  Constant_f0_7fafb/1 -> Product_c813a/2
  State_Px_2_SG_D_2_f1aec/1 -> Product_f39d7/2
  Constant_-1_1724e/1 -> Product_cb5db/1
  Product_c813a/1 -> Add_93689/1
  Product_cb5db/1 -> Divide_56a39/1
  Constant_T_w_f7f42/1 -> Divide_56a39/2
  Add_93689/1 -> Divide_8e073/1
  Constant_T_w_ec2c5/1 -> Divide_8e073/2
  Divide_56a39/1 -> Add_8d951/1
  Divide_8e073/1 -> Add_8d951/2
  Constant_T_2_bd17f/1 -> Product_e35d7/1
  Add_8d951/1 -> Product_e35d7/2
  State_Px_1_SG_D_2_41234/1 -> Add_77af2/1
  Product_f39d7/1 -> Divide_9219e/1
  Constant_T_1_cab14/1 -> Divide_9219e/2
  Add_77af2/1 -> Divide_86fee/1
  Constant_T_1_35986/1 -> Divide_86fee/2
  Divide_9219e/1 -> Add_18759/1
  Divide_86fee/1 -> Add_18759/2
  Add_18759/1 -> Blockout_d_Px_2_SG_D_2_af1ce/1

== system IEEE9Buses/SG_D_2/d_Px_3_SG_D_2_block ==
  note: d_Px_3_SG_D_2 in SG9
      | $\frac{\mathrm{Px}_{2,\mathrm{SG},D,2}+T_{4}\,\left(\frac{\mathrm{Px}_{1,\mathrm{SG},D,2}-T_{2}\,\left(\frac{\mathrm{Px}_{1,\mathrm{SG},D,2}}{T_{w}}-\frac{w_{\mathrm{SG},D,2}-2\,\pi \,f_{0}}{T_{w}}\right)}{T_{1}}-\frac{\mathrm{Px}_{2,\mathrm{SG},D,2}}{T_{1}}\right)}{T_{3}}-\frac{\mathrm{Px}_{3,\mathrm{SG},D,2}}{T_{3}}$
      | Automatically generated on 2025-09-12 21:32:42 .
  State_Px_3_SG_D_2_01548 : Inport
  State_Px_2_SG_D_2_9f207 : Inport  Port=2
  State_Px_2_SG_D_2_c3e8f : Inport  Port=3
  State_Px_1_SG_D_2_15f5c : Inport  Port=4
  State_Px_1_SG_D_2_308b2 : Inport  Port=5
  State_w_SG_D_2_e3ed6 : Inport  Port=6
  Add_51d60 : Sum
  Add_65646 : Sum
  Add_80db4 : Sum
  Add_9ec07 : Sum
  Add_b68a7 : Sum
  Add_fe765 : Sum
  Constant_-1_00f58 : Constant  Value=-1
  Constant_-1_4e29b : Constant  Value=-1
  Constant_-1_7bd45 : Constant  Value=-1
  Constant_-2.0_acb0a : Constant  Value=-2.0
  Constant_T_1_569c4 : Constant  Value=T_1
  Constant_T_1_f3dc1 : Constant  Value=T_1
  Constant_T_2_dcbc5 : Constant  Value=T_2
  Constant_T_3_59620 : Constant  Value=T_3
  Constant_T_3_82909 : Constant  Value=T_3
  Constant_T_4_3ed22 : Constant  Value=T_4
  Constant_T_w_36e10 : Constant  Value=T_w
  Constant_T_w_a2040 : Constant  Value=T_w
  Constant_f0_e6869 : Constant  Value=f0
  Constant_pi_e68e8 : Constant  Value=pi
  Divide_53037 : Product  Inputs=*/
  Divide_57344 : Product  Inputs=*/
  Divide_579dd : Product  Inputs=*/
  Divide_818fa : Product  Inputs=*/
  Divide_a224a : Product  Inputs=*/
  Divide_bf54e : Product  Inputs=*/
  Product_139de : Product
  Product_16c3d : Product
  Product_6a0bb : Product
  Product_6cf1e : Product
  Product_79e75 : Product
  Product_ae8ed : Product
  Product_c7a01 : Product
  Blockout_d_Px_3_SG_D_2_56385 : Outport
  wires:
  Constant_-2.0_acb0a/1 -> Product_6a0bb/1
  State_w_SG_D_2_e3ed6/1 -> Add_9ec07/2
  Add_80db4/1 -> Divide_579dd/1
  Constant_pi_e68e8/1 -> Product_6a0bb/2
  Constant_-1_4e29b/1 -> Product_c7a01/1
  Product_6a0bb/1 -> Product_6cf1e/1
  State_Px_2_SG_D_2_c3e8f/1 -> Product_c7a01/2
  State_Px_1_SG_D_2_308b2/1 -> Product_139de/2
  Divide_579dd/1 -> Add_65646/2
  Constant_f0_e6869/1 -> Product_6cf1e/2
  Constant_-1_00f58/1 -> Product_139de/1
  Product_6cf1e/1 -> Add_9ec07/1
  Product_139de/1 -> Divide_53037/1
  Constant_T_w_a2040/1 -> Divide_53037/2
  Divide_a224a/1 -> Add_65646/1
  Add_9ec07/1 -> Divide_818fa/1
  Product_ae8ed/1 -> Add_fe765/2
  Constant_T_w_36e10/1 -> Divide_818fa/2
  Divide_53037/1 -> Add_51d60/1
  State_Px_1_SG_D_2_15f5c/1 -> Add_fe765/1
  Divide_818fa/1 -> Add_51d60/2
  Constant_-1_7bd45/1 -> Product_16c3d/1
  Constant_T_2_dcbc5/1 -> Product_ae8ed/1
  Add_51d60/1 -> Product_ae8ed/2
  Product_c7a01/1 -> Divide_57344/1
  Constant_T_1_f3dc1/1 -> Divide_57344/2
  Add_fe765/1 -> Divide_bf54e/1
  Constant_T_1_569c4/1 -> Divide_bf54e/2
  Divide_57344/1 -> Add_b68a7/1
  Divide_bf54e/1 -> Add_b68a7/2
  Constant_T_4_3ed22/1 -> Product_79e75/1
  Add_b68a7/1 -> Product_79e75/2
  State_Px_3_SG_D_2_01548/1 -> Product_16c3d/2
  State_Px_2_SG_D_2_9f207/1 -> Add_80db4/1
  Product_79e75/1 -> Add_80db4/2
  Product_16c3d/1 -> Divide_a224a/1
  Constant_T_3_82909/1 -> Divide_a224a/2
  Constant_T_3_59620/1 -> Divide_579dd/2
  Add_65646/1 -> Blockout_d_Px_3_SG_D_2_56385/1

== system IEEE9Buses/SG_D_2/d_R_f_SG_D_2_block ==
  note: d_R_f_SG_D_2 in SG9
      | $-\frac{R_{f,\mathrm{SG},D,2}-\frac{E_{\mathrm{fd},\mathrm{SG},D,2}\,K_{F}}{T_{F}}}{T_{F}}$
      | Automatically generated on 2025-09-12 21:32:37 .
  State_E_fd_SG_D_2_fa033 : Inport
  State_R_f_SG_D_2_9e0bf : Inport  Port=2
  Constant_K_F_77fdd : Constant  Value=K_F
  Constant_T_F_45922 : Constant  Value=T_F
  Constant_T_F_92eba : Constant  Value=T_F
  Divide_4eff2 : Product  Inputs=*/
  Divide_5c8ca : Product  Inputs=*/
  Product_e900d : Product
  Subtract_c1565 : Sum  Inputs=+-
  Blockout_d_R_f_SG_D_2_1e3df : Outport
  wires:
  Constant_T_F_45922/1 -> Divide_4eff2/2
  State_E_fd_SG_D_2_fa033/1 -> Product_e900d/1
  Constant_K_F_77fdd/1 -> Product_e900d/2
  State_R_f_SG_D_2_9e0bf/1 -> Subtract_c1565/2
  Product_e900d/1 -> Divide_4eff2/1
  Divide_4eff2/1 -> Subtract_c1565/1
  Constant_T_F_92eba/1 -> Divide_5c8ca/2
  Subtract_c1565/1 -> Divide_5c8ca/1
  Divide_5c8ca/1 -> Blockout_d_R_f_SG_D_2_1e3df/1

== system IEEE9Buses/SG_D_2/d_T_m_SG_D_2_block ==
  note: d_T_m_SG_D_2 in SG9
      | $-\frac{T_{m,\mathrm{SG},D,2}-T_{0}+\frac{\mathrm{SpeedPara}\,\left(w_{\mathrm{SG},D,2}-w_{\mathrm{ref}}\right)}{2\,f_{0}\,\pi }}{T_{\mathrm{speed}}}$
      | Automatically generated on 2025-09-12 21:32:28 .
  State_w_SG_D_2_fe2e1 : Inport
  State_T_m_SG_D_2_5de5c : Inport  Port=2
  Add_7cd26 : Sum
  Add_d8e17 : Sum
  Constant_-1_81891 : Constant  Value=-1
  Constant_2.0_194af : Constant  Value=2.0
  Constant_SpeedPara_5956d : Constant  Value=SpeedPara
  Constant_T_0_96ecc : Constant  Value=T_0
  Constant_T_speed_ca3b9 : Constant  Value=T_speed
  Constant_f0_91fff : Constant  Value=f0
  Constant_pi_1c6ee : Constant  Value=pi
  Constant_w_ref_71c7d : Constant  Value=w_ref
  Divide_41f3c : Product  Inputs=*/
  Divide_5d17d : Product  Inputs=*/
  Product_3e787 : Product
  Product_53481 : Product
  Product_a5e0c : Product
  Product_dccb4 : Product
  Subtract_c4169 : Sum  Inputs=+-
  Blockout_d_T_m_SG_D_2_06e02 : Outport
  wires:
  Constant_pi_1c6ee/1 -> Product_53481/2
  Constant_-1_81891/1 -> Product_dccb4/1
  Constant_w_ref_71c7d/1 -> Add_d8e17/2
  State_w_SG_D_2_fe2e1/1 -> Product_dccb4/2
  Product_dccb4/1 -> Add_d8e17/1
  Add_7cd26/1 -> Subtract_c4169/1
  Add_d8e17/1 -> Product_3e787/2
  Constant_2.0_194af/1 -> Product_53481/1
  Constant_SpeedPara_5956d/1 -> Product_3e787/1
  Product_53481/1 -> Product_a5e0c/1
  Constant_f0_91fff/1 -> Product_a5e0c/2
  Product_3e787/1 -> Divide_41f3c/1
  Product_a5e0c/1 -> Divide_41f3c/2
  Divide_41f3c/1 -> Add_7cd26/1
  Constant_T_0_96ecc/1 -> Add_7cd26/2
  State_T_m_SG_D_2_5de5c/1 -> Subtract_c4169/2
  Subtract_c4169/1 -> Divide_5d17d/1
  Constant_T_speed_ca3b9/1 -> Divide_5d17d/2
  Divide_5d17d/1 -> Blockout_d_T_m_SG_D_2_06e02/1
